simulink model "dynamique"  (R2019b)
settings: Solver=VariableStepAuto  StartTime=0.0  StopTime=10.0  RelTol=1e-3
settings Model: Creator=Morin  LastModifiedBy=Morin

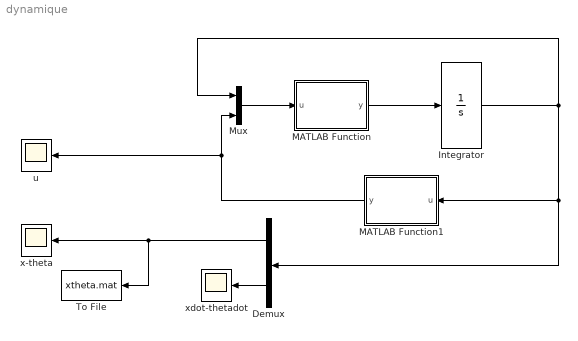
== system dynamique ==
  Demux : Demux  Outputs=2
  Integrator : Integrator
  MATLAB Function : MATLAB Function  TreatAsAtomicUnit=on
  MATLAB Function1 : MATLAB Function  TreatAsAtomicUnit=on
  Mux : Mux  Inputs=2
  To File : ToFile  Filename=xtheta.mat  SaveFormat=Timeseries
  u : Scope
  x-theta : Scope
  xdot-thetadot : Scope
  wires:
  MATLAB Function/1(y) -> Integrator/1
  Integrator/1 -> Mux/1, Demux/1, MATLAB Function1/1(u)
  Mux/1 -> MATLAB Function/1(u)
  MATLAB Function1/1(y) -> u/1, Mux/2
  Demux/1 -> To File/1, x-theta/1
  Demux/2 -> xdot-thetadot/1

== matlab function dynamique/MATLAB Function1 ==
  data: u input; y output
function y = fcn(u)

y = u;

== matlab function dynamique/MATLAB Function ==
  data: u input; y output
function y = dynamique(u)

y = u;
